simulink model "signal_conversion_sim"  (R2020b)
settings: Solver=FixedStepAuto  StartTime=0.0  StopTime=stop_time  RelTol=1e-3
InitFcn:
  | model_parameters
StopFcn:
  | verify_sim
values from neighbouring files (symbols this model uses):
  fs = audio_fs * fft_up_sample_rate    (= 6144000)    [model_parameters.m]
settings Model: Creator=t96f346  LastModifiedBy=conno
settings DataIOCC: ReturnWorkspaceOutputs=off

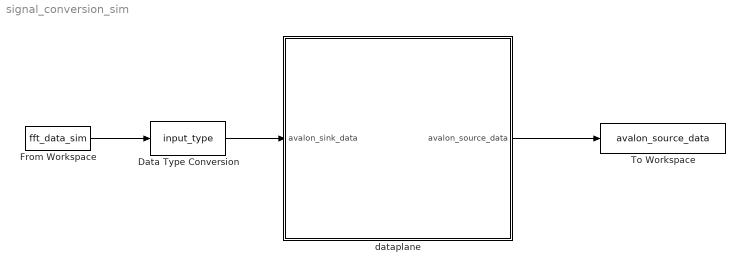
== system signal_conversion_sim ==
  Data Type Conversion : DataTypeConversion  OutDataTypeStr=input_type
  From Workspace : FromWorkspace  VariableName=fft_data_sim  SampleTime=-1  Interpolate=off  OutputAfterFinalValue=Holding final value
  To Workspace : ToWorkspace  VariableName=avalon_source_data  SampleTime=-1
  dataplane : Subsystem  TreatAsAtomicUnit=on
  wires:
  dataplane/1(avalon_source_data) -> To Workspace/1
  From Workspace/1 -> Data Type Conversion/1
  Data Type Conversion/1 -> dataplane/1(avalon_sink_data)

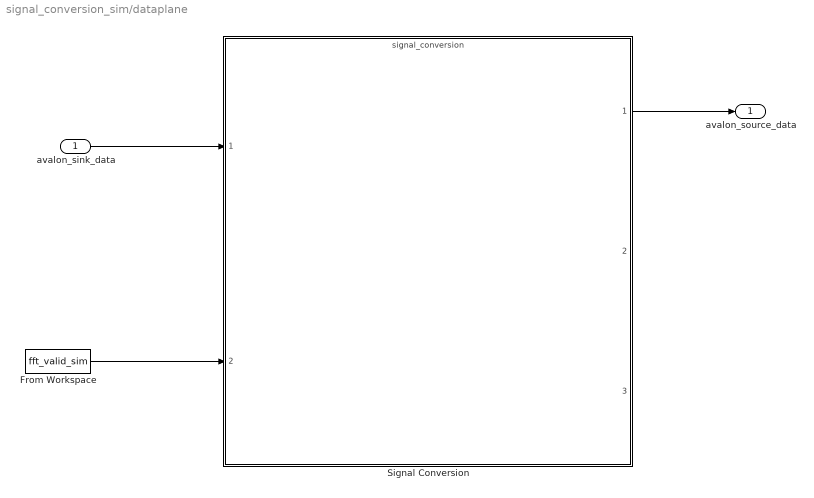
== system signal_conversion_sim/dataplane ==
  avalon_sink_data : Inport  OutDataTypeStr=input_type
  From Workspace : FromWorkspace  VariableName=fft_valid_sim  SampleTime=1/fs
  Signal Conversion : ModelReference  ModelNameDialog=signal_conversion.slx  SimulationMode=Normal  ModelReferenceVersion=1.11
  avalon_source_data : Outport  OutDataTypeStr=input_type  VectorParamsAs1DForOutWhenUnconnected=off
  wires:
  avalon_sink_data/1 -> Signal Conversion/1
  Signal Conversion/1 -> avalon_source_data/1
  From Workspace/1 -> Signal Conversion/2
